simulink model "es5oss_ACPC"  (R2022b)
settings: Solver=VariableStepAuto  StartTime=0.0  StopTime=10.0  RelTol=1e-3
values from neighbouring files (symbols this model uses):
  A = [-a b;c -d]    [ES5.m]
  B = [1;1]    [ES5.m]
  C = [1 1]    [ES5.m]
  K1 = place(A,B,avalD)    [ES5.m]
  L = place(A',C',avalO)'    [ES5.m]
  x0 = [0.5,0.3]'    [ES5.m]
settings Model: Creator=claudio  LastModifiedBy=claudio

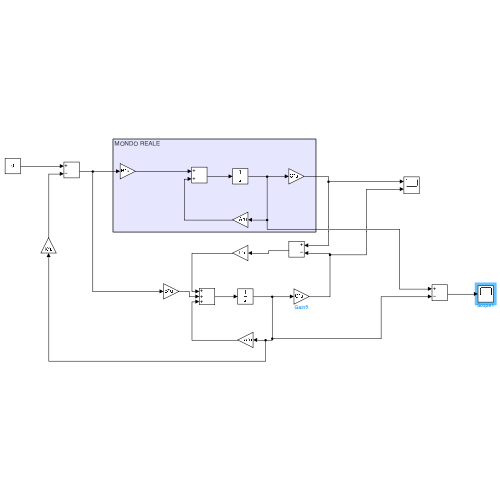
[thumbnail: Simulink's stored preview of the top-level diagram]
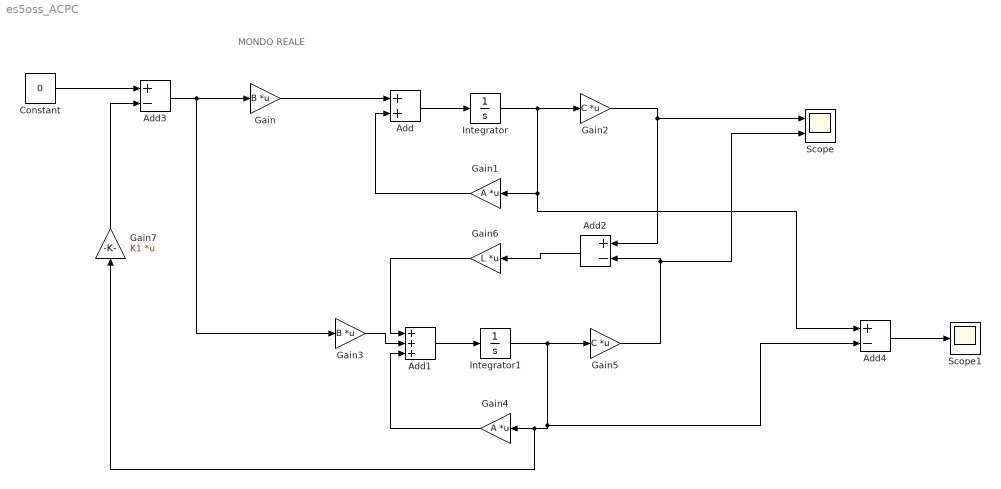
== system es5oss_ACPC ==
  note: MONDO REALE
  Add : Sum
  Add1 : Sum  Inputs=+++
  Add2 : Sum  Inputs=+-
  Add3 : Sum  Inputs=+-
  Add4 : Sum  Inputs=+-
  Constant : Constant  Value=0
  Gain : Gain  Gain=B  Multiplication=Matrix(K*u)
  Gain1 : Gain  Gain=A  Multiplication=Matrix(K*u)
  Gain2 : Gain  Gain=C  Multiplication=Matrix(K*u)
  Gain3 : Gain  Gain=B  Multiplication=Matrix(K*u)
  Gain4 : Gain  Gain=A  Multiplication=Matrix(K*u)
  Gain5 : Gain  Gain=C  Multiplication=Matrix(K*u)
  Gain6 : Gain  Gain=L  Multiplication=Matrix(K*u)
  Gain7 : Gain  Gain=K1  Multiplication=Matrix(K*u)
  Integrator : Integrator  InitialCondition=x0
  Integrator1 : Integrator
  Scope : Scope  NumInputPorts=2
  Scope1 : Scope
  wires:
  Add/1 -> Integrator/1
  Gain/1 -> Add/1
  Integrator/1 -> Add4/1, Gain1/1, Gain2/1
  Gain1/1 -> Add/2
  Integrator1/1 -> Gain5/1, Add4/2, Gain7/1, Gain4/1
  Add1/1 -> Integrator1/1
  Gain3/1 -> Add1/2
  Gain4/1 -> Add1/3
  Gain6/1 -> Add1/1
  Add2/1 -> Gain6/1
  Gain5/1 -> Scope/2, Add2/2
  Gain2/1 -> Scope/1, Add2/1
  Add3/1 -> Gain3/1, Gain/1
  Constant/1 -> Add3/1
  Gain7/1 -> Add3/2
  Add4/1 -> Scope1/1
